simulink model "PeripheralCap_Insulin37"  (R2018a)
settings: Solver=VariableStepAuto  StartTime=0.0  StopTime=10.0  RelTol=1e-3
undefined symbols (not defined in the file): Q_i_P, T_i_P, V_i_PC, V_i_PF
settings Model: Creator=cgonterman  LastModifiedBy=cgonterman

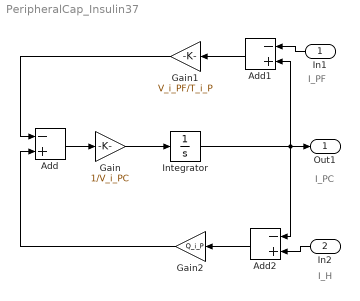
== system PeripheralCap_Insulin37 ==
  note: I_PF
  note: I_H
  note: I_PC
  In1 : Inport
  In2 : Inport  Port=2
  Add : Sum  Inputs=-+
  Add1 : Sum  Inputs=-+
  Add2 : Sum  Inputs=-+
  Gain : Gain  Gain=1/V_i_PC
  Gain1 : Gain  Gain=V_i_PF/T_i_P
  Gain2 : Gain  Gain=Q_i_P
  Integrator : Integrator
  Out1 : Outport
  wires:
  Gain/1 -> Integrator/1
  Integrator/1 -> Add1/2, Out1/1, Add2/1
  In1/1 -> Add1/1
  In2/1 -> Add2/2
  Add2/1 -> Gain2/1
  Add1/1 -> Gain1/1
  Gain1/1 -> Add/1
  Gain2/1 -> Add/2
  Add/1 -> Gain/1
